simulink model "PD_gravity_compensation"  (R2017b)
settings: Solver=FixedStepAuto  StartTime=0.0  StopTime=100  FixedStep=0.1  RelTol=1e-3
values from neighbouring files (symbols this model uses):
  kd = 5    [PD_gravity_compensation_init.m]    (also in inverse_dynamics_init.m)
  kp = 2    [PD_gravity_compensation_init.m]    (also in inverse_dynamics_init.m = 3)
  q_desired = [pi/4,3*pi/4,0,3*pi/4,-pi/4,-3*pi/4]    [PD_gravity_compensation_init.m]    (also in inverse_dynamics_init.m = [pi,pi/4,-pi,0,pi/4,0]; robot_initial_config.m = p560.ikine6s(TTCP_World_desired))
  qd_lower_sat_limit = -5    [PD_gravity_compensation_init.m]    (also in inverse_dynamics_init.m)
  qd_upper_sat_limit = 5    [PD_gravity_compensation_init.m]    (also in inverse_dynamics_init.m)
undefined symbols (not defined in the file or in its folder): p560, slcoulomb
libraries: roblocks x1
settings Model: Creator=albertllebariafabrias  LastModifiedBy=guillecasado

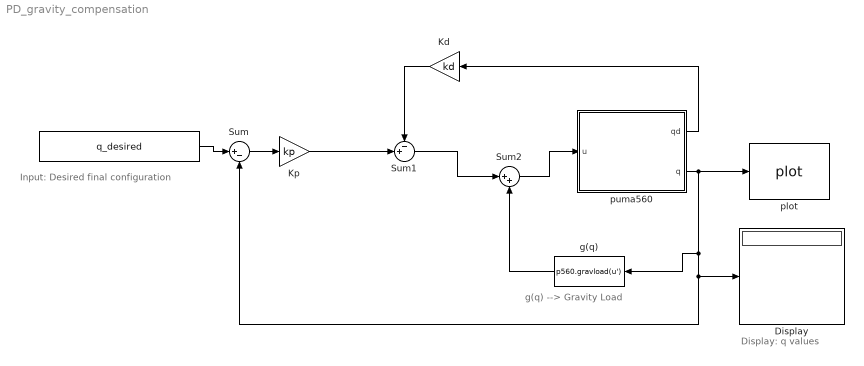
== system PD_gravity_compensation ==
  note: g(q) --> Gravity Load
  note: Display: q values
  note: Input: Desired final configuration
  " " : Constant  Value=q_desired
  Display : Display
  Kd : Gain  Gain=kd
  Kp : Gain  Gain=kp
  Sum : Sum  Inputs=|+-
  Sum1 : Sum  Inputs=-+|
  Sum2 : Sum  Inputs=|++
  g(q) : MATLABFcn  MATLABFcn=p560.gravload(u')
  plot : roblocks/Arm/plot  robot=p560  fps=fps  holdplot=on
  puma560 : Subsystem
  wires:
  Sum/1 -> Kp/1
  Kp/1 -> Sum1/2
  Kd/1 -> Sum1/1
  puma560/1(qd) -> Kd/1
  puma560/2(q) -> plot/1, g(q)/1, Display/1, Sum/2
  g(q)/1 -> Sum2/2
  " "/1 -> Sum/1
  Sum1/1 -> Sum2/1
  Sum2/1 -> puma560/1(u)

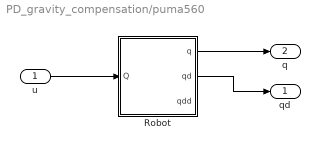
== system PD_gravity_compensation/puma560 ==
  u : Inport
  Robot : Subsystem  AncestorBlock=roblocks/Arm/Robot  mask{robot=p560, q0=[0,0,0,0,0,0]}
      mask prompts: robot "Robot object"; q0 "Initial state"
      mask help: Rigid-body dynamic model of robot.
      mask init:
      | if isa(robot, 'SerialLink')
      |     rname = robot.name;
      |     %fprintf('**robot name is %s\n', rname);
      | else
      |     rname = '';
      |     n = 0
      | end
      mask Help:
      | Simulates the forward (direct) rigid-body dynamics of the robot described
      | by the given robot object.  For given applied joint torque/force it computes
      | the instaneous joint coordinates, velocities and acclerations.
      | 
      | 
      | <b>Parameters::</b>
      | 
      | robot (SerialLink) a dynamic model of an N-link serial link manipulator
      | q0 (1xN)  Initial joint coordinates
      | 
      | <b>Inputs::</b>
      | 
      | Q (1xN) the generalized joint force (torque or force) required to achieve
      | the motion state (q, qd, qdd).
      | 
      | <b>Outputs::</b>
      | 
      | q (1xN) joint coordinates
      | qd (1xN) joint coordinate velocity
      | qdd (1xN) joint coordinate acceleration
      | 
      | 
      | <b>Notes::</b>
      | 
      | - Required to simulate robot rigid body motion.
      | - Implemented using the recursive Newton-Euler scheme (RNE).
      | - A wrapper for the Toolbox method accel() which in turn depends on the
      |   method rne().
      mask Display:
      | port_label('input', 1, 'Q')
      | port_label('output', 1, 'q')
      | port_label('output', 2, 'qd')
      | port_label('output', 3, 'qdd')
      | text(0.1, 0.9,  rname, 'horizontalAlignment', 'left')
  qd : Outport
  q : Outport  Port=2
  wires:
  u/1 -> Robot/1(Q)
  Robot/1(q) -> q/1
  Robot/2(qd) -> qd/1

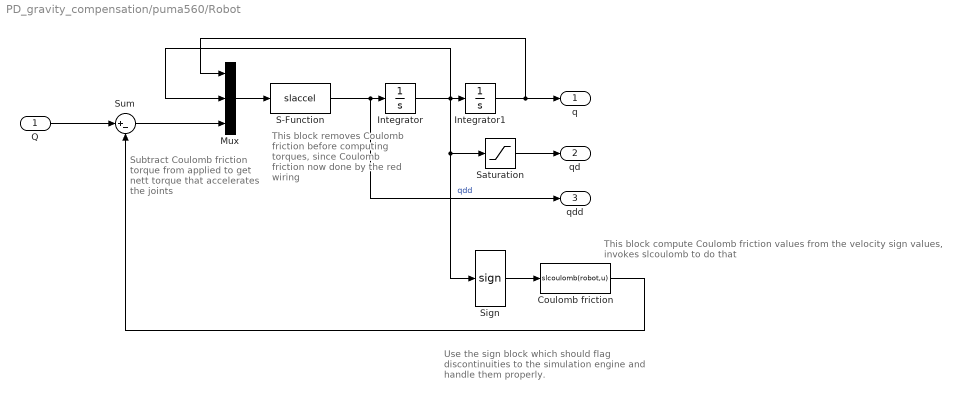
== system PD_gravity_compensation/puma560/Robot ==
  note: This block removes Coulomb friction before computing torques, since Coulomb friction now done by the red wiring
  note: Subtract Coulomb friction torque from applied to get nett torque that accelerates the joints
  note: This block compute Coulomb friction values from the velocity sign values, invokes slcoulomb to do that
  note: Use the sign block which should flag discontinuities to the simulation engine and
      | handle them properly.
  Q : Inport
  Coulomb friction : MATLABFcn  MATLABFcn=slcoulomb(robot,u)  OutputDimensions=[robot.n 1]  Output1D=off
  Integrator : Integrator
  Integrator1 : Integrator  InitialCondition=q0
  Mux : Mux  Inputs=3
  S-Function : S-Function  FunctionName=slaccel  Parameters=robot.nofriction()  SFunctionDeploymentMode=off  EnableBusSupport=off
  Saturation : Saturate  UpperLimit=qd_upper_sat_limit  LowerLimit=qd_lower_sat_limit  ZeroCross=off
  Sign : Signum
  Sum : Sum  Inputs=|+-
  q : Outport
  qd : Outport  Port=2
  qdd : Outport  Port=3
  wires:
  S-Function/1 -> qdd/1, Integrator/1  "qdd"
  Mux/1 -> S-Function/1
  Integrator/1 -> Sign/1, Saturation/1, Integrator1/1, Mux/2
  Q/1 -> Sum/1
  Sum/1 -> Mux/3
  Coulomb friction/1 -> Sum/2
  Sign/1 -> Coulomb friction/1
  Saturation/1 -> qd/1
  Integrator1/1 -> q/1, Mux/1
